simulink model "AuM_HA_05_Vorlage_A1"  (R2022a)
settings: Solver=VariableStepAuto  StartTime=0.0  StopTime=5  FixedStep=1e-8  MaxStep=1e-4  MinStep=1e-9  RelTol=1e-9  EnableMultiTasking=on
values from neighbouring files (symbols this model uses):
  J = 450e-6    (= 0.00045)    [AuM_HA05_Parameter_Synchronmaschine_ARW_q_d.m]
  L_S = 4e-3    (= 0.004)    [AuM_HA05_Parameter_Synchronmaschine_ARW_q_d.m]
  p = 5    [AuM_HA05_Parameter_Synchronmaschine_ARW_q_d.m]
  Psi_P = 4.5e-3    (= 0.0045)    [AuM_HA05_Parameter_Synchronmaschine_ARW_q_d.m]
  R_S = 0.58    [AuM_HA05_Parameter_Synchronmaschine_ARW_q_d.m]
  T_S = L_S/R_S    (= 0.00689655172414)    [AuM_HA05_Parameter_Synchronmaschine_ARW_q_d.m]
  U_d = 24    [AuM_HA05_Parameter_Synchronmaschine_ARW_q_d.m]
settings Model: Creator=junglas  LastModifiedBy=Gianluca
settings SolverCC: MaxConsecutiveZCs=10000  ZeroCrossAlgorithm=Adaptive  AlgebraicLoopSolver=TrustRegion
settings DataIOCC: ReturnWorkspaceOutputs=off
settings OptimizationCC: LifeSpan=inf
settings DebuggingCC: UnconnectedInputMsg=warning  UnconnectedOutputMsg=warning  UnconnectedLineMsg=warning  SFUnexpectedBacktrackingDiag=warning  SFNoUnconditionalDefaultTransitionDiag=warning  SFExecutionAtInitializationDiag=none  SFMachineParentedDataDiag=warning  ArithmeticOperatorsInVariantConditions=warning
settings SFSimCC: SimUseLocalCustomCode=off  CustomCodeUndefinedFunction=UseInterfaceOnly
settings RTWCC: RTWUseLocalCustomCode=off
settings CodeAppCC: StateflowObjectComments=on
settings GRTTargetCC: TargetLangStandard=C89/C90 (ANSI)
settings ConfigComp: CovMetricSettings=dw  CovSaveCumulativeToWorkspaceVar=on  CovSaveSingleToWorkspaceVar=on  CovExternalEMLEnable=off

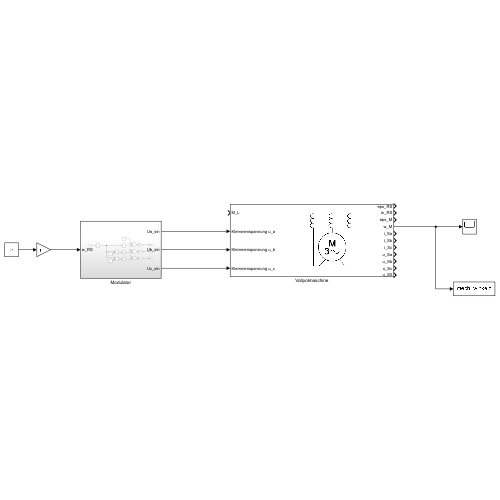
[thumbnail: Simulink's stored preview of the top-level diagram]
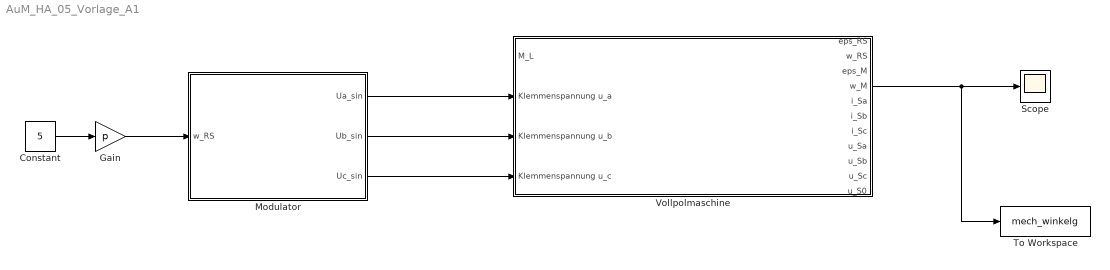
== system AuM_HA_05_Vorlage_A1 ==
  Constant : Constant  Value=5
  Gain : Gain  Gain=p
  Modulator : Subsystem
  Scope : Scope
  To Workspace : ToWorkspace  VariableName=mech_winkelg  SaveFormat=Timeseries  SampleTime=-1
  Vollpolmaschine : Subsystem
      mask Display: image('Motor_Symbol.png'); % Use "Edit Image" on toolstrip to change.
  wires:
  Modulator/1(Ua_sin) -> Vollpolmaschine/2(Klemmenspannung u_a)
  Modulator/2(Ub_sin) -> Vollpolmaschine/3(Klemmenspannung u_b)
  Modulator/3(Uc_sin) -> Vollpolmaschine/4(Klemmenspannung u_c)
  Constant/1 -> Gain/1
  Gain/1 -> Modulator/1(w_RS)
  Vollpolmaschine/4(w_M) -> To Workspace/1, Scope/1

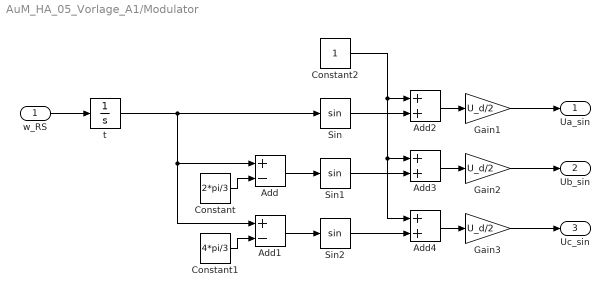
== system AuM_HA_05_Vorlage_A1/Modulator ==
  w_RS : Inport
  Add : Sum  Inputs=+-
  Add1 : Sum  Inputs=+-
  Add2 : Sum
  Add3 : Sum
  Add4 : Sum
  Constant : Constant  Value=2*pi/3
  Constant1 : Constant  Value=4*pi/3
  Constant2 : Constant
  Gain1 : Gain  Gain=U_d/2
  Gain2 : Gain  Gain=U_d/2
  Gain3 : Gain  Gain=U_d/2
  Sin : Trigonometry
  Sin1 : Trigonometry
  Sin2 : Trigonometry
  t : Integrator
  Ua_sin : Outport
  Ub_sin : Outport  Port=2
  Uc_sin : Outport  Port=3
  wires:
  Sin/1 -> Add2/2
  Gain1/1 -> Ua_sin/1
  Add1/1 -> Sin2/1
  Gain3/1 -> Uc_sin/1
  Sin2/1 -> Add4/2
  Sin1/1 -> Add3/2
  Constant2/1 -> Add4/1, Add3/1, Add2/1
  Add3/1 -> Gain2/1
  Add2/1 -> Gain1/1
  t/1 -> Add1/1, Add/1, Sin/1
  Constant1/1 -> Add1/2
  Add4/1 -> Gain3/1
  Constant/1 -> Add/2
  Add/1 -> Sin1/1
  Gain2/1 -> Ub_sin/1
  w_RS/1 -> t/1

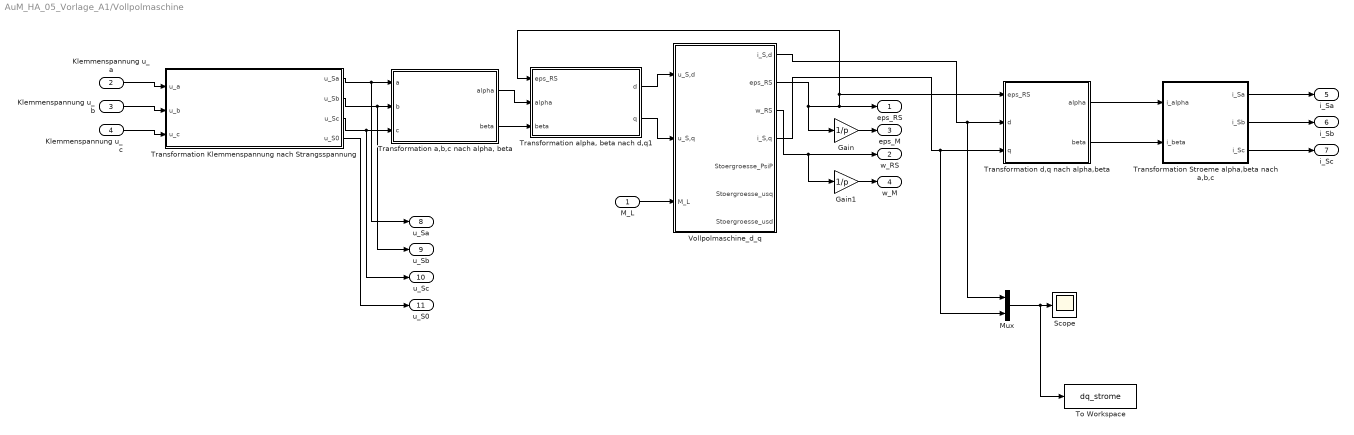
== system AuM_HA_05_Vorlage_A1/Vollpolmaschine ==
  M_L : Inport
  Klemmenspannung u_a : Inport  Port=2
  Klemmenspannung u_b : Inport  Port=3
  Klemmenspannung u_c : Inport  Port=4
  Gain : Gain  Gain=1/p
  Gain1 : Gain  Gain=1/p
  Mux : Mux  Inputs=2
  Scope : Scope
  To Workspace : ToWorkspace  VariableName=dq_strome  SaveFormat=Timeseries  SampleTime=-1
  Transformation Klemmenspannung nach Strangsspannung : MATLAB Function  TreatAsAtomicUnit=on
  Transformation Stroeme alpha,beta nach a,b,c : MATLAB Function  TreatAsAtomicUnit=on
  "Transformation a,b,c nach alpha, beta" : MATLAB Function  TreatAsAtomicUnit=on
  "Transformation alpha, beta nach d,q1" : MATLAB Function  TreatAsAtomicUnit=on
  Transformation d,q nach alpha,beta : MATLAB Function  TreatAsAtomicUnit=on
  Vollpolmaschine_d_q : Subsystem
  eps_RS : Outport  VectorParamsAs1DForOutWhenUnconnected=off
  w_RS : Outport  Port=2  VectorParamsAs1DForOutWhenUnconnected=off
  eps_M : Outport  Port=3  VectorParamsAs1DForOutWhenUnconnected=off
  w_M : Outport  Port=4  VectorParamsAs1DForOutWhenUnconnected=off
  i_Sa : Outport  Port=5  VectorParamsAs1DForOutWhenUnconnected=off
  i_Sb : Outport  Port=6  VectorParamsAs1DForOutWhenUnconnected=off
  i_Sc : Outport  Port=7  VectorParamsAs1DForOutWhenUnconnected=off
  u_Sa : Outport  Port=8  VectorParamsAs1DForOutWhenUnconnected=off
  u_Sb : Outport  Port=9  VectorParamsAs1DForOutWhenUnconnected=off
  u_Sc : Outport  Port=10  VectorParamsAs1DForOutWhenUnconnected=off
  u_S0 : Outport  Port=11  VectorParamsAs1DForOutWhenUnconnected=off
  wires:
  Transformation Klemmenspannung nach Strangsspannung/4(u_S0) -> u_S0/1
  Transformation Stroeme alpha,beta nach a,b,c/3(i_Sc) -> i_Sc/1
  Transformation Stroeme alpha,beta nach a,b,c/2(i_Sb) -> i_Sb/1
  Transformation Stroeme alpha,beta nach a,b,c/1(i_Sa) -> i_Sa/1
  Transformation d,q nach alpha,beta/2(beta) -> Transformation Stroeme alpha,beta nach a,b,c/2(i_beta)
  Transformation d,q nach alpha,beta/1(alpha) -> Transformation Stroeme alpha,beta nach a,b,c/1(i_alpha)
  "Transformation alpha, beta nach d,q1"/1(d) -> Vollpolmaschine_d_q/1(u_S,d)
  Gain1/1 -> w_M/1
  Gain/1 -> eps_M/1
  Klemmenspannung u_c/1 -> Transformation Klemmenspannung nach Strangsspannung/3(u_c)
  Klemmenspannung u_b/1 -> Transformation Klemmenspannung nach Strangsspannung/2(u_b)
  Klemmenspannung u_a/1 -> Transformation Klemmenspannung nach Strangsspannung/1(u_a)
  "Transformation alpha, beta nach d,q1"/2(q) -> Vollpolmaschine_d_q/2(u_S,q)
  "Transformation a,b,c nach alpha, beta"/2(beta) -> "Transformation alpha, beta nach d,q1"/3(beta)
  "Transformation a,b,c nach alpha, beta"/1(alpha) -> "Transformation alpha, beta nach d,q1"/2(alpha)
  M_L/1 -> Vollpolmaschine_d_q/3(M_L)
  Transformation Klemmenspannung nach Strangsspannung/3(u_Sc) -> u_Sc/1, "Transformation a,b,c nach alpha, beta"/3(c)
  Vollpolmaschine_d_q/2(eps_RS) -> Gain/1, "Transformation alpha, beta nach d,q1"/1(eps_RS), Transformation d,q nach alpha,beta/1(eps_RS), eps_RS/1
  Transformation Klemmenspannung nach Strangsspannung/1(u_Sa) -> "Transformation a,b,c nach alpha, beta"/1(a), u_Sa/1
  Vollpolmaschine_d_q/3(w_RS) -> w_RS/1, Gain1/1
  Transformation Klemmenspannung nach Strangsspannung/2(u_Sb) -> "Transformation a,b,c nach alpha, beta"/2(b), u_Sb/1
  Vollpolmaschine_d_q/1(i_S,d) -> Transformation d,q nach alpha,beta/2(d), Mux/1
  Vollpolmaschine_d_q/4(i_S,q) -> Transformation d,q nach alpha,beta/3(q), Mux/2
  Mux/1 -> To Workspace/1, Scope/1

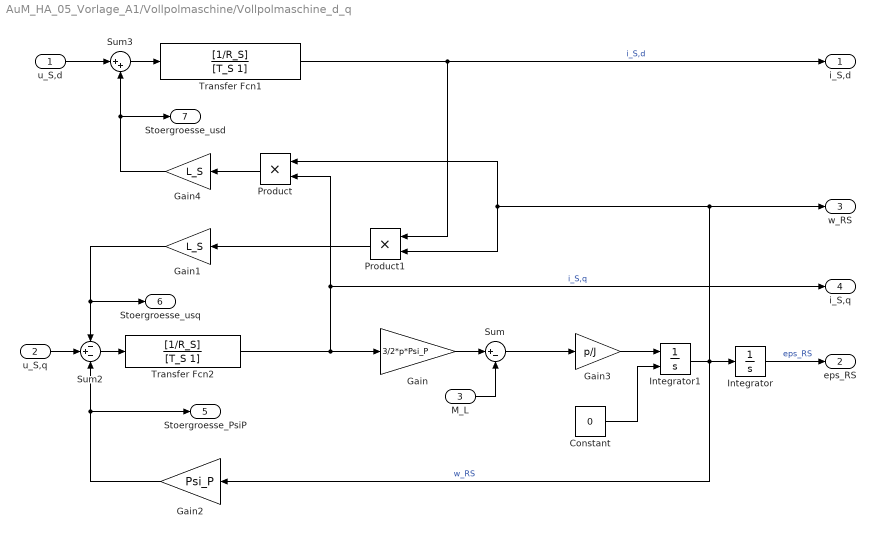
== system AuM_HA_05_Vorlage_A1/Vollpolmaschine/Vollpolmaschine_d_q ==
  u_S,d : Inport
  u_S,q : Inport  Port=2
  M_L : Inport  Port=3
  Constant : Constant  Value=0
  Gain : Gain  Gain=3/2*p*Psi_P
  Gain1 : Gain  Gain=L_S
  Gain2 : Gain  Gain=Psi_P
  Gain3 : Gain  Gain=p/J
  Gain4 : Gain  Gain=L_S
  Integrator : Integrator
  Integrator1 : Integrator  InitialConditionSource=external
  Product : Product
  Product1 : Product
  Sum : Sum  Inputs=|+-
  Sum2 : Sum  Inputs=-+-
  Sum3 : Sum  Inputs=|++
  Transfer Fcn1 : TransferFcn  Numerator=[1/R_S]  Denominator=[T_S 1]
  Transfer Fcn2 : TransferFcn  Numerator=[1/R_S]  Denominator=[T_S 1]
  i_S,d : Outport  VectorParamsAs1DForOutWhenUnconnected=off
  eps_RS : Outport  Port=2  VectorParamsAs1DForOutWhenUnconnected=off
  w_RS : Outport  Port=3  VectorParamsAs1DForOutWhenUnconnected=off
  i_S,q : Outport  Port=4  VectorParamsAs1DForOutWhenUnconnected=off
  Stoergroesse_PsiP : Outport  Port=5  VectorParamsAs1DForOutWhenUnconnected=off
  Stoergroesse_usq : Outport  Port=6  VectorParamsAs1DForOutWhenUnconnected=off
  Stoergroesse_usd : Outport  Port=7  VectorParamsAs1DForOutWhenUnconnected=off
  wires:
  Constant/1 -> Integrator1/2
  Transfer Fcn2/1 -> Product/2, i_S,q/1, Gain/1  "i_S,q"
  Gain4/1 -> Sum3/2, Stoergroesse_usd/1
  u_S,d/1 -> Sum3/1
  Gain1/1 -> Sum2/1, Stoergroesse_usq/1
  u_S,q/1 -> Sum2/2
  Product1/1 -> Gain1/1
  Transfer Fcn1/1 -> Product1/1, i_S,d/1  "i_S,d"
  Product/1 -> Gain4/1
  Sum3/1 -> Transfer Fcn1/1
  Gain2/1 -> Sum2/3, Stoergroesse_PsiP/1
  Gain3/1 -> Integrator1/1
  Gain/1 -> Sum/1
  M_L/1 -> Sum/2
  Sum/1 -> Gain3/1
  Integrator/1 -> eps_RS/1  "eps_RS"
  Integrator1/1 -> Gain2/1, Product1/2, Product/1, w_RS/1, Integrator/1  "w_RS"
  Sum2/1 -> Transfer Fcn2/1

== matlab function AuM_HA_05_Vorlage_A1/Vollpolmaschine/Transformation Klemmenspannung nach Strangsspannung ==
  data: u_a input; u_Sa output; u_b input; u_c input; u_Sb output; u_Sc output; u_S0 output
function [u_Sa,u_Sb,u_Sc,u_S0] = fcn(u_a,u_b,u_c)
%Konvertiert Klemmenspannungen in Strangspannungen
u_S0=u_a/3+u_b/3+u_c/3;
u_Sa=u_a-u_S0;
u_Sb=u_b-u_S0;
u_Sc=u_c-u_S0;
end

== matlab function AuM_HA_05_Vorlage_A1/Vollpolmaschine/Transformation Stroeme alpha,beta nach a,b,c ==
  data: i_alpha input; i_Sa output; i_beta input; i_Sb output; i_Sc output
function [i_Sa,i_Sb,i_Sc] = fcn(i_alpha,i_beta)
i_Sa=i_alpha;
i_Sb=-1/2*i_alpha+sqrt(3)/2*i_beta;
i_Sc=-i_Sa-i_Sb;

== matlab function AuM_HA_05_Vorlage_A1/Vollpolmaschine/Transformation a,b,c nach alpha, beta ==
  data: a input; alpha output; b input; c input; beta output
 function [alpha,beta] = fcn(a,b,c)
alpha=2/3*(a+cos(2*pi/2)*b+cos(4*pi/3)*c);
beta=2/3*(sin(2*pi/3)*b+sin(4*pi/3)*c);

== matlab function AuM_HA_05_Vorlage_A1/Vollpolmaschine/Transformation alpha, beta nach d,q1 ==
  data: eps_RS input; d output; alpha input; beta input; q output
function [d,q] = fcn(eps_RS,alpha,beta)
d=cos(eps_RS)*alpha+sin(eps_RS)*beta;
q=-sin(eps_RS)*alpha+cos(eps_RS)*beta;

== matlab function AuM_HA_05_Vorlage_A1/Vollpolmaschine/Transformation d,q nach alpha,beta ==
  data: eps_RS input; alpha output; d input; q input; beta output
function [alpha,beta] = fcn(eps_RS,d,q)
alpha=cos(eps_RS)*d-sin(eps_RS)*q;
beta=sin(eps_RS)*d+cos(eps_RS)*q;
